simulink model "Monorail_Auxiliary_Power_Unit"  (R2021b)
settings: Solver=ode1  StartTime=0.0  StopTime=2.00  FixedStep=1e-06  MaxStep=1e-4  RelTol=1e-3
InitFcn:
  | %Input
  | V_supply_max = 910;
  | V_supply_min = 490;
  | V_supply_nom = 750;
  | R_supply = 1e-06;
  | L_in = 0.5e-03;
  | C_in = 215e-06;
  | R_Precharge = 1;
  | 
  | %PSFB_Voltage_Control
  | t_psfb_on = 0.05;
  | f_sw = 10e03;
  | V_dc_ref = 700;
  | V_dc_init = 450;
  | V_bat_ref = 24;
  | V_bat_init = 14;
  | Count_prd = 5000;
  | Half_prd = 2500;
  | Half_prd_fix = 2700;
  | Half_prd_var = 2300;
  | t_softstart = 100e-03;
  | Scale_factor_High = 1/737;
  | Scale_factor_Low = 1/48;
  | Kp_psfb = 2;
  | Ki_psfb =20;
  | Kp_feed = 0.00001;
  | PI_max = 1;
  | PI_min = 0;
  | t_enable = 1e-03;
  | Dead_prd = 1e-03
  | 
  | %PSFB_Current_Control
  | Scale_factor_i = 1/800;
  | I_cnst = 450;
  | I_over = 460;
  | Kp_psfb_i = 10;
  | Ki_psfb_i = 20;
  | 
  | %HF_Transformer
  | P_txf = 50e03;
  | f_txf = 10e03;
  | V_pri_txf = 1e03;
  | V_sec_high_txf = 720;
  | V_sec_low_txf = 27;
  | 
  | %DC_Link
  | L_filt = 1e-03;
  | C_filt = 215e-06;
  | R_Bleeder_700V = 0.5e03;
  | R_Bleeder_24V = 1e03
  | 
  | %Inverter_Control
  | t_inv_on = 1.5;
  | f_fund = 50;
  | V_phase_ref = 240;
  | Scale_factor_inv = 1/50e03;
  | Kp_inv = 0.05;
  | Ki_inv = 0.1;
  | PI_inv_max = 1;
  | PI_inv_min = -1;
  | ... (+27 lines)
undefined symbols (not defined in the file): Ion, Lithium
libraries: spsSeriesRLCBranchLib x35, spsIGBTDiodeLib x14, spsDiodeLib x13, spsMeanLib x11, spsBreakerLib x9, spsVoltageMeasurementLib x9, simulink x8, spsRMSLib x8, spsCurrentMeasurementLib x6, dspfdesign x6, spsabctodq0Lib x4, spsLinearTransformerLib x2
(part 3 of 3)

== system Monorail_Auxiliary_Power_Unit/Second Stage/Pulse Generator/Pulse/SVGEN_DQ/Switching Time Calculation/If Action Subsystem7 ==
  In1 : Inport
  Action Port : ActionPort  ActionPortLabel=elseif(u1==2 | u1==5)
  Add : Sum
  Demux : Demux  Outputs=3
  Gain : Gain  Gain=-1
  Mux : Mux  Inputs=3
  Out1 : Outport
  wires:
  In1/1 -> Demux/1
  Demux/2 -> Add/1
  Demux/3 -> Add/2
  Mux/1 -> Out1/1
  Add/1 -> Mux/1
  Demux/1 -> Gain/1, Mux/2
  Gain/1 -> Mux/3

== system Monorail_Auxiliary_Power_Unit/Second Stage/Pulse Generator/Pulse/SVGEN_DQ/Switching Time Calculation/If Action Subsystem8 ==
  In1 : Inport
  Action Port : ActionPort  ActionPortLabel=else
  Add : Sum
  Demux : Demux  Outputs=3
  Gain : Gain  Gain=-1
  Gain1 : Gain  Gain=-1
  Mux : Mux  Inputs=3
  Out1 : Outport
  wires:
  In1/1 -> Demux/1
  Mux/1 -> Out1/1
  Demux/3 -> Mux/1, Gain/1
  Gain/1 -> Mux/2
  Gain1/1 -> Mux/3
  Add/1 -> Gain1/1
  Demux/1 -> Add/1
  Demux/2 -> Add/2

== system Monorail_Auxiliary_Power_Unit/Second Stage/Pulse Generator/Voltage Loop/V PI Block/PI_MACRO (for 0)/If Action Subsystem1 ==
  In1 : Inport
  Action Port : ActionPort  ActionPortLabel=if(u1 == u2)
  Out1 : Outport
  wires:
  In1/1 -> Out1/1

== system Monorail_Auxiliary_Power_Unit/Second Stage/Pulse Generator/Voltage Loop/V PI Block/PI_MACRO (for 0)/If Action Subsystem3 ==
  In1 : Inport
  Action Port : ActionPort  ActionPortLabel=else
  Out1 : Outport
  wires:
  In1/1 -> Out1/1

== system Monorail_Auxiliary_Power_Unit/Second Stage/Pulse Generator/Voltage Loop/V PI Block/PI_MACRO (for D)/If Action Subsystem1 ==
  In1 : Inport
  Action Port : ActionPort  ActionPortLabel=if(u1 == u2)
  Out1 : Outport
  wires:
  In1/1 -> Out1/1

== system Monorail_Auxiliary_Power_Unit/Second Stage/Pulse Generator/Voltage Loop/V PI Block/PI_MACRO (for D)/If Action Subsystem3 ==
  In1 : Inport
  Action Port : ActionPort  ActionPortLabel=else
  Out1 : Outport
  wires:
  In1/1 -> Out1/1

== system Monorail_Auxiliary_Power_Unit/Second Stage/Pulse Generator/Voltage Loop/V PI Block/PI_MACRO (for Q)/If Action Subsystem1 ==
  In1 : Inport
  Action Port : ActionPort  ActionPortLabel=if(u1 == u2)
  Out1 : Outport
  wires:
  In1/1 -> Out1/1

== system Monorail_Auxiliary_Power_Unit/Second Stage/Pulse Generator/Voltage Loop/V PI Block/PI_MACRO (for Q)/If Action Subsystem3 ==
  In1 : Inport
  Action Port : ActionPort  ActionPortLabel=else
  Out1 : Outport
  wires:
  In1/1 -> Out1/1
